simulink model "IEEE14_case"  (R2024b)
settings: Solver=FixedStepAuto  StartTime=0  StopTime=2  FixedStep=1e-7  RelTol=1e-3
values from neighbouring files (symbols this model uses):
  GFL_15_Bva = 0.009    [IEEE14_parameters.m]
  GFL_15_C_bus_pu = 7.179419    [IEEE14_parameters.m]
  GFL_15_f0 = 60    [IEEE14_parameters.m]
  GFL_15_I_id = 691.26967    [IEEE14_parameters.m]
  GFL_15_I_iq = 691.26967    [IEEE14_parameters.m]
  GFL_15_I_od = 45.2207    [IEEE14_parameters.m]
  GFL_15_I_oq = 45.2207    [IEEE14_parameters.m]
  GFL_15_I_pll = 0.78    [IEEE14_parameters.m]
  GFL_15_Kdi = 0.09    [IEEE14_parameters.m]
  GFL_15_Kdo = 0.9    [IEEE14_parameters.m]
  GFL_15_Kqi = 0.09    [IEEE14_parameters.m]
  GFL_15_Kqo = 0.9    [IEEE14_parameters.m]
  GFL_15_Lg_pu = 0.631447    [IEEE14_parameters.m]
  GFL_15_mode = 1    [IEEE14_parameters.m]
  GFL_15_P_id = 3.7166    [IEEE14_parameters.m]
  GFL_15_P_iq = 3.7166    [IEEE14_parameters.m]
  GFL_15_P_od = 0.4798    [IEEE14_parameters.m]
  GFL_15_P_oq = 0.4798    [IEEE14_parameters.m]
  GFL_15_P_pll = 290.42    [IEEE14_parameters.m]
  GFL_15_Qe_ref = 0.2    [IEEE14_parameters.m]
  GFL_15_Rg_pu = 0.024016    [IEEE14_parameters.m]
  GFL_15_Sbase = 1.000000e+4    (= 10000)    [IEEE14_parameters.m]
  GFL_15_Tdi = 0.01    [IEEE14_parameters.m]
  GFL_15_Tdo = 0.2    [IEEE14_parameters.m]
  GFL_15_Tqi = 0.01    [IEEE14_parameters.m]
  GFL_15_Tqo = 0.2    [IEEE14_parameters.m]
  GFL_15_Vbase = 380    [IEEE14_parameters.m]
  GFL_15_Vdc_ref = 1.011475    [IEEE14_parameters.m]
  GFL_15_Vdcbase = 700    [IEEE14_parameters.m]
  GFL_15_vq_ref = 0    [IEEE14_parameters.m]
  GFL_16_Bva = 0.002    [IEEE14_parameters.m]
  GFL_16_C_bus_pu = 7.179419    [IEEE14_parameters.m]
  GFL_16_f0 = 60    [IEEE14_parameters.m]
  GFL_16_I_id = 691.26967    [IEEE14_parameters.m]
  GFL_16_I_iq = 691.26967    [IEEE14_parameters.m]
  GFL_16_I_od = 45.2207    [IEEE14_parameters.m]
  GFL_16_I_oq = 45.2207    [IEEE14_parameters.m]
  GFL_16_I_pll = 0.78    [IEEE14_parameters.m]
  GFL_16_Kdi = 0.05    [IEEE14_parameters.m]
  GFL_16_Kdo = 0.5    [IEEE14_parameters.m]
  GFL_16_Kqi = 0.05    [IEEE14_parameters.m]
  GFL_16_Kqo = 0.5    [IEEE14_parameters.m]
  GFL_16_Lg_pu = 0.631447    [IEEE14_parameters.m]
  GFL_16_mode = 1    [IEEE14_parameters.m]
  GFL_16_P_id = 3.7166    [IEEE14_parameters.m]
  GFL_16_P_iq = 3.7166    [IEEE14_parameters.m]
  GFL_16_P_od = 0.4798    [IEEE14_parameters.m]
  GFL_16_P_oq = 0.4798    [IEEE14_parameters.m]
  GFL_16_P_pll = 290.42    [IEEE14_parameters.m]
  GFL_16_Qe_ref = 0.2    [IEEE14_parameters.m]
  GFL_16_Rg_pu = 0.024016    [IEEE14_parameters.m]
  GFL_16_Sbase = 1.000000e+4    (= 10000)    [IEEE14_parameters.m]
  GFL_16_Tdi = 0.01    [IEEE14_parameters.m]
  GFL_16_Tdo = 0.2    [IEEE14_parameters.m]
  GFL_16_Tqi = 0.01    [IEEE14_parameters.m]
  GFL_16_Tqo = 0.2    [IEEE14_parameters.m]
  GFL_16_Vbase = 380    [IEEE14_parameters.m]
  GFL_16_Vdc_ref = 1.01144    [IEEE14_parameters.m]
  GFL_16_Vdcbase = 700    [IEEE14_parameters.m]
  GFL_16_vq_ref = 0    [IEEE14_parameters.m]
  GFL_17_Bva = 0.002    [IEEE14_parameters.m]
  GFL_17_C_bus_pu = 7.179419    [IEEE14_parameters.m]
  GFL_17_f0 = 60    [IEEE14_parameters.m]
  GFL_17_I_id = 691.26967    [IEEE14_parameters.m]
  GFL_17_I_iq = 691.26967    [IEEE14_parameters.m]
  GFL_17_I_od = 45.2207    [IEEE14_parameters.m]
  GFL_17_I_oq = 45.2207    [IEEE14_parameters.m]
  GFL_17_I_pll = 0.78    [IEEE14_parameters.m]
  GFL_17_Kdi = 0.05    [IEEE14_parameters.m]
  GFL_17_Kdo = 0.5    [IEEE14_parameters.m]
  GFL_17_Kqi = 0.05    [IEEE14_parameters.m]
  GFL_17_Kqo = 0.5    [IEEE14_parameters.m]
  GFL_17_Lg_pu = 0.631447    [IEEE14_parameters.m]
  GFL_17_mode = 1    [IEEE14_parameters.m]
  GFL_17_P_id = 3.7166    [IEEE14_parameters.m]
  GFL_17_P_iq = 3.7166    [IEEE14_parameters.m]
  GFL_17_P_od = 0.4798    [IEEE14_parameters.m]
  GFL_17_P_oq = 0.4798    [IEEE14_parameters.m]
  GFL_17_P_pll = 290.42    [IEEE14_parameters.m]
  GFL_17_Qe_ref = 0.2    [IEEE14_parameters.m]
  GFL_17_Rg_pu = 0.024016    [IEEE14_parameters.m]
  GFL_17_Sbase = 1.000000e+4    (= 10000)    [IEEE14_parameters.m]
  GFL_17_Tdi = 0.01    [IEEE14_parameters.m]
  GFL_17_Tdo = 0.2    [IEEE14_parameters.m]
  GFL_17_Tqi = 0.01    [IEEE14_parameters.m]
  GFL_17_Tqo = 0.2    [IEEE14_parameters.m]
  GFL_17_Vbase = 380    [IEEE14_parameters.m]
  GFL_17_Vdc_ref = 1.011632    [IEEE14_parameters.m]
  GFL_17_Vdcbase = 700    [IEEE14_parameters.m]
  GFL_17_vq_ref = 0    [IEEE14_parameters.m]
  GFL_18_Bva = 0.002    [IEEE14_parameters.m]
  GFL_18_C_bus_pu = 7.179419    [IEEE14_parameters.m]
  GFL_18_f0 = 60    [IEEE14_parameters.m]
  GFL_18_I_id = 691.26967    [IEEE14_parameters.m]
  GFL_18_I_iq = 691.26967    [IEEE14_parameters.m]
  GFL_18_I_od = 45.2207    [IEEE14_parameters.m]
  GFL_18_I_oq = 45.2207    [IEEE14_parameters.m]
  GFL_18_I_pll = 0.78    [IEEE14_parameters.m]
  GFL_18_Kdi = 0.05    [IEEE14_parameters.m]
  GFL_18_Kdo = 0.5    [IEEE14_parameters.m]
  GFL_18_Kqi = 0.05    [IEEE14_parameters.m]
  GFL_18_Kqo = 0.5    [IEEE14_parameters.m]
  GFL_18_Lg_pu = 0.631447    [IEEE14_parameters.m]
  GFL_18_mode = 1    [IEEE14_parameters.m]
  GFL_18_P_id = 3.7166    [IEEE14_parameters.m]
  GFL_18_P_iq = 3.7166    [IEEE14_parameters.m]
  GFL_18_P_od = 0.4798    [IEEE14_parameters.m]
  GFL_18_P_oq = 0.4798    [IEEE14_parameters.m]
  GFL_18_P_pll = 290.42    [IEEE14_parameters.m]
  GFL_18_Qe_ref = 0.2    [IEEE14_parameters.m]
  GFL_18_Rg_pu = 0.024016    [IEEE14_parameters.m]
  GFL_18_Sbase = 1.000000e+4    (= 10000)    [IEEE14_parameters.m]
  GFL_18_Tdi = 0.01    [IEEE14_parameters.m]
  GFL_18_Tdo = 0.2    [IEEE14_parameters.m]
  GFL_18_Tqi = 0.01    [IEEE14_parameters.m]
  GFL_18_Tqo = 0.2    [IEEE14_parameters.m]
  GFL_18_Vbase = 380    [IEEE14_parameters.m]
  GFL_18_Vdc_ref = 1.011572    [IEEE14_parameters.m]
  GFL_18_Vdcbase = 700    [IEEE14_parameters.m]
  GFL_18_vq_ref = 0    [IEEE14_parameters.m]
  ... (+180 more)
(part 18 of 25)

== system IEEE14_case/SG_D_2/d_psi_fd_SG_D_2_block ==
  note: d_psi_fd_SG_D_2 in case14gfl
      | $-\frac{\psi _{\mathrm{fd},\mathrm{SG},D,2}-E_{\mathrm{fd},\mathrm{SG},D,2}+\left(x_{d}-x_{\mathrm{dd}}\right)\,\left(\frac{\frac{\psi _{\mathrm{1d},\mathrm{SG},D,2}\,\left(x_{\mathrm{dd}}-x_{\mathrm{ddd}}\right)}{x_{\mathrm{dd}}-x_{l}}-\psi _{d,\mathrm{SG},D,2}+\frac{\psi _{\mathrm{fd},\mathrm{SG},D,2}\,\left(x_{\mathrm{ddd}}-x_{l}\right)}{x_{\mathrm{dd}}-x_{l}}}{x_{\mathrm{ddd}}}-\frac{\left(x_{\mathrm{dd}}-x_{\mathrm{ddd}}\right)\,\left(\psi _{\mathrm{1d},\mathrm{SG},D,2}-\psi _{\mathrm{fd},\mathrm{SG},D,2}+\frac{\left(x_{\mathrm{dd}}-x_{l}\right)\,\left(\frac{\psi _{\mathrm{1d},\mathrm{SG},D,2}\,\left(x_{\mathrm{dd}}-x_{\mathrm{ddd}}\right)}{x_{\mathrm{dd}}-x_{l}}-\psi _{d,\mathrm{SG},D,2}+\frac{\psi _{\mathrm{fd},\mathrm{SG},D,2}\,\left(x_{\mathrm{ddd}}-x_{l}\right)}{x_{\mathrm{dd}}-x_{l}}\right)}{x_{\mathrm{ddd}}}\right)}{{\left(x_{\mathrm{dd}}-x_{l}\right)}^2}\right)}{T_{\mathrm{dd}}}$
      | Automatically generated on 2025-10-09 21:30:57 .
  State_E_fd_SG_D_2_01a4d : Inport
  State_psi_fd_SG_D_2_2df35 : Inport  Port=2
  State_psi_1d_SG_D_2_84bab : Inport  Port=3
  State_psi_fd_SG_D_2_f521e : Inport  Port=4
  State_psi_1d_SG_D_2_c8d78 : Inport  Port=5
  State_psi_d_SG_D_2_1798b : Inport  Port=6
  State_psi_fd_SG_D_2_82c24 : Inport  Port=7
  State_psi_1d_SG_D_2_e893c : Inport  Port=8
  State_psi_d_SG_D_2_c30ab : Inport  Port=9
  State_psi_fd_SG_D_2_fdcf2 : Inport  Port=10
  Add_3611d : Sum
  Add_4026f : Sum
  Constant_-1_921ca : Constant  Value=-1
  Constant_-1_96da0 : Constant  Value=-1
  Constant_-1_d9610 : Constant  Value=-1
  Constant_2.0_a7520 : Constant  Value=2.0
  Constant_T_dd_003d2 : Constant  Value=T_dd
  Constant_x_d_08df9 : Constant  Value=x_d
  Constant_x_dd_19849 : Constant  Value=x_dd
  Constant_x_dd_47a17 : Constant  Value=x_dd
  Constant_x_dd_565fe : Constant  Value=x_dd
  Constant_x_dd_6360d : Constant  Value=x_dd
  Constant_x_dd_6ee8d : Constant  Value=x_dd
  Constant_x_dd_aa39f : Constant  Value=x_dd
  Constant_x_dd_b6005 : Constant  Value=x_dd
  Constant_x_dd_bbfae : Constant  Value=x_dd
  Constant_x_dd_de48f : Constant  Value=x_dd
  Constant_x_dd_e38b5 : Constant  Value=x_dd
  Constant_x_ddd_0bd47 : Constant  Value=x_ddd
  Constant_x_ddd_846c0 : Constant  Value=x_ddd
  Constant_x_ddd_a248a : Constant  Value=x_ddd
  Constant_x_ddd_a406a : Constant  Value=x_ddd
  Constant_x_ddd_bb480 : Constant  Value=x_ddd
  Constant_x_ddd_ca766 : Constant  Value=x_ddd
  Constant_x_ddd_d5431 : Constant  Value=x_ddd
  Constant_x_l_1bf20 : Constant  Value=x_l
  Constant_x_l_31a91 : Constant  Value=x_l
  Constant_x_l_34653 : Constant  Value=x_l
  Constant_x_l_4eace : Constant  Value=x_l
  Constant_x_l_5aec2 : Constant  Value=x_l
  Constant_x_l_a09cf : Constant  Value=x_l
  Constant_x_l_a2996 : Constant  Value=x_l
  Constant_x_l_ed53a : Constant  Value=x_l
  Divide_1a091 : Product  Inputs=*/
  Divide_320e0 : Product  Inputs=*/
  Divide_4596a : Product  Inputs=*/
  Divide_604a6 : Product  Inputs=*/
  Divide_730ee : Product  Inputs=*/
  Divide_7d69b : Product  Inputs=*/
  Divide_a9374 : Product  Inputs=*/
  Divide_c19ec : Product  Inputs=*/
  Power_098d0 : Math  Operator=pow
  Product_03136 : Product
  Product_07e41 : Product
  Product_25612 : Product
  Product_42463 : Product
  Product_6e0f0 : Product
  Product_8a094 : Product
  Product_90eff : Product
  Product_9aa8a : Product
  Product_a124e : Product
  Product_f461e : Product
  Subtract_04977 : Sum  Inputs=+-
  Subtract_04bd0 : Sum  Inputs=+-
  Subtract_05140 : Sum  Inputs=+-
  Subtract_185b4 : Sum  Inputs=+-
  Subtract_2504d : Sum  Inputs=+-
  Subtract_3f8c2 : Sum  Inputs=+-
  Subtract_446d6 : Sum  Inputs=+-
  Subtract_4df95 : Sum  Inputs=+-
  Subtract_639b5 : Sum  Inputs=+-
  Subtract_64a07 : Sum  Inputs=+-
  Subtract_745c1 : Sum  Inputs=+-
  Subtract_8dab0 : Sum  Inputs=+-
  Subtract_a59fc : Sum  Inputs=+-
  Subtract_ab7fc : Sum  Inputs=+-
  Subtract_cb1a9 : Sum  Inputs=+-
  Subtract_cd5af : Sum  Inputs=+-
  Subtract_cde08 : Sum  Inputs=+-
  Subtract_d078d : Sum  Inputs=+-
  Subtract_ebb1a : Sum  Inputs=+-
  Blockout_d_psi_fd_SG_D_2_ab69d : Outport
  wires:
  Constant_x_dd_bbfae/1 -> Subtract_4df95/1
  Constant_-1_96da0/1 -> Product_42463/1
  Constant_x_l_a09cf/1 -> Subtract_d078d/2
  Divide_1a091/1 -> Add_3611d/1
  Subtract_745c1/1 -> Product_25612/2
  Constant_x_l_1bf20/1 -> Subtract_4df95/2
  Product_25612/1 -> Divide_730ee/1
  State_psi_1d_SG_D_2_c8d78/1 -> Product_42463/2
  Constant_x_dd_b6005/1 -> Subtract_64a07/1
  Product_6e0f0/1 -> Divide_1a091/1
  Constant_x_dd_aa39f/1 -> Subtract_cde08/1
  Constant_x_ddd_d5431/1 -> Subtract_64a07/2
  Constant_x_dd_47a17/1 -> Subtract_8dab0/1
  Product_42463/1 -> Product_f461e/1
  Subtract_64a07/1 -> Product_f461e/2
  State_psi_d_SG_D_2_c30ab/1 -> Add_3611d/2
  Constant_x_ddd_0bd47/1 -> Subtract_745c1/1
  Constant_x_l_31a91/1 -> Subtract_745c1/2
  Product_f461e/1 -> Divide_a9374/1
  Subtract_4df95/1 -> Divide_a9374/2
  State_psi_fd_SG_D_2_82c24/1 -> Product_25612/1
  Subtract_04977/1 -> Product_8a094/2
  Constant_x_dd_565fe/1 -> Subtract_ab7fc/1
  Constant_x_l_34653/1 -> Subtract_ab7fc/2
  Product_07e41/1 -> Product_8a094/1
  Divide_a9374/1 -> Add_4026f/1
  State_psi_d_SG_D_2_1798b/1 -> Add_4026f/2
  Subtract_ab7fc/1 -> Divide_730ee/2
  Constant_x_dd_e38b5/1 -> Subtract_d078d/1
  Constant_x_ddd_a248a/1 -> Subtract_cd5af/1
  Add_4026f/1 -> Subtract_2504d/1
  Divide_730ee/1 -> Subtract_2504d/2
  Constant_-1_d9610/1 -> Product_a124e/1
  Product_9aa8a/1 -> Divide_4596a/1
  State_psi_1d_SG_D_2_e893c/1 -> Product_a124e/2
  Subtract_cde08/1 -> Product_07e41/2
  Constant_x_dd_19849/1 -> Subtract_05140/1
  Divide_4596a/1 -> Subtract_a59fc/2
  Constant_-1_921ca/1 -> Product_07e41/1
  Constant_x_ddd_ca766/1 -> Subtract_05140/2
  Constant_x_ddd_a406a/1 -> Divide_7d69b/2
  Subtract_d078d/1 -> Product_03136/1
  Subtract_2504d/1 -> Product_03136/2
  State_psi_fd_SG_D_2_f521e/1 -> Subtract_ebb1a/2
  Product_a124e/1 -> Product_6e0f0/1
  Subtract_05140/1 -> Product_6e0f0/2
  Constant_2.0_a7520/1 -> Power_098d0/2
  State_psi_1d_SG_D_2_84bab/1 -> Subtract_ebb1a/1
  Constant_x_dd_de48f/1 -> Subtract_639b5/1
  Subtract_cd5af/1 -> Product_9aa8a/2
  Constant_x_l_5aec2/1 -> Subtract_639b5/2
  Constant_x_l_a2996/1 -> Subtract_cd5af/2
  Constant_x_ddd_bb480/1 -> Subtract_cde08/2
  Subtract_8dab0/1 -> Divide_4596a/2
  Product_03136/1 -> Divide_7d69b/1
  Subtract_639b5/1 -> Divide_1a091/2
  State_psi_fd_SG_D_2_fdcf2/1 -> Product_9aa8a/1
  Constant_x_l_4eace/1 -> Subtract_8dab0/2
  Constant_x_dd_6ee8d/1 -> Subtract_185b4/1
  Subtract_ebb1a/1 -> Subtract_04977/1
  Divide_7d69b/1 -> Subtract_04977/2
  Constant_x_l_ed53a/1 -> Subtract_185b4/2
  Subtract_185b4/1 -> Power_098d0/1
  Add_3611d/1 -> Subtract_a59fc/1
  Product_8a094/1 -> Divide_320e0/1
  Power_098d0/1 -> Divide_320e0/2
  Subtract_a59fc/1 -> Divide_c19ec/1
  Constant_x_ddd_846c0/1 -> Divide_c19ec/2
  Constant_x_d_08df9/1 -> Subtract_cb1a9/1
  Constant_x_dd_6360d/1 -> Subtract_cb1a9/2
  Divide_320e0/1 -> Subtract_3f8c2/1
  Divide_c19ec/1 -> Subtract_3f8c2/2
  State_E_fd_SG_D_2_01a4d/1 -> Subtract_446d6/1
  State_psi_fd_SG_D_2_2df35/1 -> Subtract_446d6/2
  Subtract_cb1a9/1 -> Product_90eff/1
  Subtract_3f8c2/1 -> Product_90eff/2
  Subtract_446d6/1 -> Subtract_04bd0/1
  Product_90eff/1 -> Subtract_04bd0/2
  Subtract_04bd0/1 -> Divide_604a6/1
  Constant_T_dd_003d2/1 -> Divide_604a6/2
  Divide_604a6/1 -> Blockout_d_psi_fd_SG_D_2_ab69d/1

== system IEEE14_case/SG_D_2/d_psi_gq_SG_D_2_block ==
  note: d_psi_gq_SG_D_2 in case14gfl
      | $-\frac{\psi _{\mathrm{gq},\mathrm{SG},D,2}+\left(x_{q}-x_{\mathrm{qd}}\right)\,\left(\frac{\psi _{q,\mathrm{SG},D,2}+\frac{\psi _{\mathrm{gq},\mathrm{SG},D,2}\,\left(x_{l}-x_{\mathrm{qdd}}\right)}{x_{l}-x_{\mathrm{qd}}}+\frac{\psi _{\mathrm{kq},\mathrm{SG},D,2}\,\left(x_{\mathrm{qd}}-x_{\mathrm{qdd}}\right)}{x_{l}-x_{\mathrm{qd}}}}{x_{\mathrm{qdd}}}+\frac{\left(x_{\mathrm{qd}}-x_{\mathrm{qdd}}\right)\,\left(\psi _{\mathrm{gq},\mathrm{SG},D,2}+\psi _{\mathrm{kq},\mathrm{SG},D,2}+\frac{\left(x_{l}-x_{\mathrm{qd}}\right)\,\left(\psi _{q,\mathrm{SG},D,2}+\frac{\psi _{\mathrm{gq},\mathrm{SG},D,2}\,\left(x_{l}-x_{\mathrm{qdd}}\right)}{x_{l}-x_{\mathrm{qd}}}+\frac{\psi _{\mathrm{kq},\mathrm{SG},D,2}\,\left(x_{\mathrm{qd}}-x_{\mathrm{qdd}}\right)}{x_{l}-x_{\mathrm{qd}}}\right)}{x_{\mathrm{qdd}}}\right)}{{\left(x_{l}-x_{\mathrm{qd}}\right)}^2}\right)}{T_{\mathrm{qd}}}$
      | Automatically generated on 2025-10-09 21:31:05 .
  State_psi_gq_SG_D_2_f404a : Inport
  State_psi_gq_SG_D_2_79e41 : Inport  Port=2
  State_psi_kq_SG_D_2_229b6 : Inport  Port=3
  State_psi_gq_SG_D_2_41ece : Inport  Port=4
  State_psi_kq_SG_D_2_a4801 : Inport  Port=5
  State_psi_q_SG_D_2_c887c : Inport  Port=6
  State_psi_gq_SG_D_2_c13c7 : Inport  Port=7
  State_psi_kq_SG_D_2_c4824 : Inport  Port=8
  State_psi_q_SG_D_2_400a1 : Inport  Port=9
  Add_2b762 : Sum
  Add_5087b : Sum
  Add_8326a : Sum
  Add_a2ab4 : Sum
  Add_a58ef : Sum
  Add_b9338 : Sum
  Add_bad94 : Sum
  Add_c4542 : Sum
  Add_e5a10 : Sum
  Add_ea486 : Sum
  Add_f567a : Sum
  Add_f8f87 : Sum
  Constant_-1_15cd5 : Constant  Value=-1
  Constant_-1_69318 : Constant  Value=-1
  Constant_-1_75525 : Constant  Value=-1
  Constant_-1_8ad9f : Constant  Value=-1
  Constant_-1_a28c5 : Constant  Value=-1
  Constant_-1_ae299 : Constant  Value=-1
  Constant_-1_b65de : Constant  Value=-1
  Constant_-1_d519c : Constant  Value=-1
  Constant_-1_e17b9 : Constant  Value=-1
  Constant_-1_efabb : Constant  Value=-1
  Constant_2.0_97bc5 : Constant  Value=2.0
  Constant_T_qd_686ff : Constant  Value=T_qd
  Constant_x_l_09c66 : Constant  Value=x_l
  Constant_x_l_1d2f7 : Constant  Value=x_l
  Constant_x_l_4d818 : Constant  Value=x_l
  Constant_x_l_57d53 : Constant  Value=x_l
  Constant_x_l_74c75 : Constant  Value=x_l
  Constant_x_l_b1845 : Constant  Value=x_l
  Constant_x_l_ba1dd : Constant  Value=x_l
  Constant_x_l_bbcc9 : Constant  Value=x_l
  Constant_x_q_f52e3 : Constant  Value=x_q
  Constant_x_qd_2dcf1 : Constant  Value=x_qd
  Constant_x_qd_3806a : Constant  Value=x_qd
  Constant_x_qd_3a214 : Constant  Value=x_qd
  Constant_x_qd_46c49 : Constant  Value=x_qd
  Constant_x_qd_478ae : Constant  Value=x_qd
  Constant_x_qd_63b72 : Constant  Value=x_qd
  Constant_x_qd_820ca : Constant  Value=x_qd
  Constant_x_qd_9db90 : Constant  Value=x_qd
  Constant_x_qd_b7357 : Constant  Value=x_qd
  Constant_x_qd_e39da : Constant  Value=x_qd
  Constant_x_qdd_17fcd : Constant  Value=x_qdd
  Constant_x_qdd_4d231 : Constant  Value=x_qdd
  Constant_x_qdd_b2109 : Constant  Value=x_qdd
  Constant_x_qdd_b62fd : Constant  Value=x_qdd
  Constant_x_qdd_bd892 : Constant  Value=x_qdd
  Constant_x_qdd_c0bf7 : Constant  Value=x_qdd
  Constant_x_qdd_c1908 : Constant  Value=x_qdd
  Divide_500ab : Product  Inputs=*/
  Divide_5990b : Product  Inputs=*/
  Divide_60d9c : Product  Inputs=*/
  Divide_8a86b : Product  Inputs=*/
  Divide_97166 : Product  Inputs=*/
  Divide_a2283 : Product  Inputs=*/
  Divide_d0dda : Product  Inputs=*/
  Divide_f3509 : Product  Inputs=*/
  Power_100eb : Math  Operator=pow
  Product_2ab9d : Product
  Product_2ef50 : Product
  Product_52ea3 : Product
  Product_6e281 : Product
  Product_94fc7 : Product
  Product_9831b : Product
  Product_9d28f : Product
  Product_a2030 : Product
  Product_aac4e : Product
  Product_ac00d : Product
  Product_acce0 : Product
  Product_b35c4 : Product
  Product_b7c07 : Product
  Product_c4254 : Product
  Product_e9acb : Product
  Product_ef741 : Product
  Product_f98fe : Product
  Subtract_18ab3 : Sum  Inputs=+-
  Subtract_23d70 : Sum  Inputs=+-
  Subtract_3e5e5 : Sum  Inputs=+-
  Subtract_52e88 : Sum  Inputs=+-
  Subtract_71078 : Sum  Inputs=+-
  Subtract_881b9 : Sum  Inputs=+-
  Subtract_c6265 : Sum  Inputs=+-
  Subtract_cf1d4 : Sum  Inputs=+-
  Blockout_d_psi_gq_SG_D_2_f3eae : Outport
  wires:
  Constant_x_l_b1845/1 -> Product_52ea3/2
  Constant_x_l_57d53/1 -> Product_acce0/2
  Constant_x_qd_2dcf1/1 -> Subtract_881b9/1
  Constant_x_l_ba1dd/1 -> Product_a2030/2
  Constant_x_qdd_17fcd/1 -> Subtract_71078/2
  Constant_-1_ae299/1 -> Product_b35c4/1
  Constant_-1_e17b9/1 -> Product_aac4e/1
  State_psi_gq_SG_D_2_79e41/1 -> Add_8326a/1
  Constant_x_qdd_c0bf7/1 -> Subtract_881b9/2
  Constant_x_qd_b7357/1 -> Subtract_71078/1
  Constant_x_l_bbcc9/1 -> Product_b35c4/2
  Constant_x_l_09c66/1 -> Product_aac4e/2
  Product_b35c4/1 -> Add_c4542/1
  Product_aac4e/1 -> Add_2b762/1
  Constant_x_l_74c75/1 -> Product_94fc7/2
  Constant_x_l_1d2f7/1 -> Product_ac00d/2
  Constant_x_qd_3806a/1 -> Add_c4542/2
  Constant_x_qdd_bd892/1 -> Add_2b762/2
  Constant_-1_15cd5/1 -> Product_94fc7/1
  Constant_x_qd_820ca/1 -> Add_ea486/2
  Constant_x_qdd_b62fd/1 -> Add_a58ef/2
  State_psi_gq_SG_D_2_41ece/1 -> Product_2ef50/1
  Add_c4542/1 -> Divide_500ab/2
  Add_2b762/1 -> Product_2ef50/2
  Constant_x_qd_46c49/1 -> Subtract_23d70/2
  Product_94fc7/1 -> Add_5087b/1
  Constant_x_qd_3a214/1 -> Add_5087b/2
  State_psi_kq_SG_D_2_a4801/1 -> Product_ef741/1
  Divide_97166/1 -> Subtract_cf1d4/1
  Subtract_881b9/1 -> Product_ef741/2
  Product_2ef50/1 -> Divide_97166/1
  Add_5087b/1 -> Divide_97166/2
  Add_e5a10/1 -> Product_9d28f/2
  Product_ef741/1 -> Divide_500ab/1
  Constant_-1_8ad9f/1 -> Product_ac00d/1
  Divide_500ab/1 -> Subtract_cf1d4/2
  Constant_-1_69318/1 -> Product_52ea3/1
  Constant_-1_a28c5/1 -> Product_acce0/1
  Product_ac00d/1 -> Add_bad94/1
  Constant_x_qdd_4d231/1 -> Subtract_52e88/2
  Constant_x_qd_63b72/1 -> Add_bad94/2
  Subtract_cf1d4/1 -> Add_e5a10/1
  Constant_-1_b65de/1 -> Product_a2030/1
  State_psi_q_SG_D_2_c887c/1 -> Add_e5a10/2
  Product_52ea3/1 -> Add_ea486/1
  Product_acce0/1 -> Add_a58ef/1
  Constant_-1_75525/1 -> Product_9831b/1
  Product_9d28f/1 -> Divide_d0dda/1
  Constant_x_l_4d818/1 -> Product_9831b/2
  Product_2ab9d/1 -> Add_f567a/2
  Constant_x_qd_e39da/1 -> Subtract_52e88/1
  Add_bad94/1 -> Product_9d28f/1
  State_psi_gq_SG_D_2_c13c7/1 -> Product_e9acb/1
  Add_ea486/1 -> Divide_f3509/2
  Add_a58ef/1 -> Product_e9acb/2
  Product_9831b/1 -> Add_b9338/1
  Constant_x_qd_478ae/1 -> Add_b9338/2
  State_psi_kq_SG_D_2_c4824/1 -> Product_f98fe/1
  Subtract_52e88/1 -> Product_f98fe/2
  Divide_f3509/1 -> Subtract_18ab3/2
  State_psi_kq_SG_D_2_229b6/1 -> Add_8326a/2
  Product_f98fe/1 -> Divide_f3509/1
  Constant_x_qdd_c1908/1 -> Divide_d0dda/2
  Product_e9acb/1 -> Divide_8a86b/1
  Add_b9338/1 -> Divide_8a86b/2
  Constant_-1_d519c/1 -> Product_6e281/1
  Subtract_71078/1 -> Product_6e281/2
  Add_8326a/1 -> Subtract_3e5e5/1
  Divide_d0dda/1 -> Subtract_3e5e5/2
  Product_a2030/1 -> Add_a2ab4/1
  Constant_x_qd_9db90/1 -> Add_a2ab4/2
  Divide_8a86b/1 -> Subtract_18ab3/1
  Product_6e281/1 -> Product_b7c07/1
  Subtract_3e5e5/1 -> Product_b7c07/2
  Add_a2ab4/1 -> Power_100eb/1
  Constant_2.0_97bc5/1 -> Power_100eb/2
  Subtract_18ab3/1 -> Add_f8f87/1
  State_psi_q_SG_D_2_400a1/1 -> Add_f8f87/2
  Product_b7c07/1 -> Divide_a2283/1
  Power_100eb/1 -> Divide_a2283/2
  Add_f8f87/1 -> Divide_60d9c/1
  Constant_x_qdd_b2109/1 -> Divide_60d9c/2
  Constant_x_q_f52e3/1 -> Subtract_23d70/1
  Divide_a2283/1 -> Subtract_c6265/1
  Divide_60d9c/1 -> Subtract_c6265/2
  Divide_5990b/1 -> Blockout_d_psi_gq_SG_D_2_f3eae/1
  Constant_-1_efabb/1 -> Product_c4254/1
  State_psi_gq_SG_D_2_f404a/1 -> Product_c4254/2
  Subtract_23d70/1 -> Product_2ab9d/1
  Subtract_c6265/1 -> Product_2ab9d/2
  Product_c4254/1 -> Add_f567a/1
  Add_f567a/1 -> Divide_5990b/1
  Constant_T_qd_686ff/1 -> Divide_5990b/2

== system IEEE14_case/SG_D_2/d_psi_kq_SG_D_2_block ==
  note: d_psi_kq_SG_D_2 in case14gfl
      | $-\frac{\psi _{\mathrm{gq},\mathrm{SG},D,2}+\psi _{\mathrm{kq},\mathrm{SG},D,2}+\frac{\left(x_{l}-x_{\mathrm{qd}}\right)\,\left(\psi _{q,\mathrm{SG},D,2}+\frac{\psi _{\mathrm{gq},\mathrm{SG},D,2}\,\left(x_{l}-x_{\mathrm{qdd}}\right)}{x_{l}-x_{\mathrm{qd}}}+\frac{\psi _{\mathrm{kq},\mathrm{SG},D,2}\,\left(x_{\mathrm{qd}}-x_{\mathrm{qdd}}\right)}{x_{l}-x_{\mathrm{qd}}}\right)}{x_{\mathrm{qdd}}}}{T_{\mathrm{qdd}}}$
      | Automatically generated on 2025-10-09 21:31:07 .
  State_psi_gq_SG_D_2_f92a1 : Inport
  State_psi_kq_SG_D_2_f7bb1 : Inport  Port=2
  State_psi_gq_SG_D_2_cbe5c : Inport  Port=3
  State_psi_kq_SG_D_2_18fe7 : Inport  Port=4
  State_psi_q_SG_D_2_cfb7c : Inport  Port=5
  Add_2481c : Sum
  Add_2fdb3 : Sum
  Add_3b297 : Sum
  Add_3ce2d : Sum
  Add_7fdac : Sum
  Add_eb29d : Sum
  Constant_-1_13a81 : Constant  Value=-1
  Constant_-1_44d95 : Constant  Value=-1
  Constant_-1_6f5fa : Constant  Value=-1
  Constant_-1_e2c15 : Constant  Value=-1
  Constant_-1_e723b : Constant  Value=-1
  Constant_T_qdd_cc972 : Constant  Value=T_qdd
  Constant_x_l_9fa0f : Constant  Value=x_l
  Constant_x_l_c253f : Constant  Value=x_l
  Constant_x_l_dc0da : Constant  Value=x_l
  Constant_x_l_e4987 : Constant  Value=x_l
  Constant_x_qd_849ec : Constant  Value=x_qd
  Constant_x_qd_9b99b : Constant  Value=x_qd
  Constant_x_qd_a0e14 : Constant  Value=x_qd
  Constant_x_qd_a3048 : Constant  Value=x_qd
  Constant_x_qdd_317d9 : Constant  Value=x_qdd
  Constant_x_qdd_60f94 : Constant  Value=x_qdd
  Constant_x_qdd_dadcf : Constant  Value=x_qdd
  Divide_2b384 : Product  Inputs=*/
  Divide_80f05 : Product  Inputs=*/
  Divide_847ec : Product  Inputs=*/
  Divide_c48ac : Product  Inputs=*/
  Product_39d4f : Product
  Product_45e1e : Product
  Product_6192a : Product
  Product_87c85 : Product
  Product_998de : Product
  Product_a46e6 : Product
  Product_adb8e : Product
  Product_e290e : Product
  Subtract_b28c8 : Sum  Inputs=+-
  Subtract_b9688 : Sum  Inputs=+-
  Subtract_d8af5 : Sum  Inputs=+-
  Blockout_d_psi_kq_SG_D_2_03e6e : Outport
  wires:
  State_psi_kq_SG_D_2_f7bb1/1 -> Subtract_b9688/2
  Constant_-1_44d95/1 -> Product_6192a/1
  Constant_-1_e2c15/1 -> Product_e290e/1
  Constant_x_l_e4987/1 -> Product_e290e/2
  Constant_x_qdd_317d9/1 -> Add_2fdb3/2
  Constant_x_l_c253f/1 -> Product_6192a/2
  Constant_x_qd_a3048/1 -> Subtract_b28c8/1
  Constant_T_qdd_cc972/1 -> Divide_c48ac/2
  Constant_-1_13a81/1 -> Product_45e1e/1
  Product_e290e/1 -> Add_2fdb3/1
  Constant_x_qdd_dadcf/1 -> Subtract_b28c8/2
  Constant_x_l_9fa0f/1 -> Product_45e1e/2
  Divide_c48ac/1 -> Blockout_d_psi_kq_SG_D_2_03e6e/1
  State_psi_gq_SG_D_2_cbe5c/1 -> Product_39d4f/1
  Add_2fdb3/1 -> Product_39d4f/2
  Product_6192a/1 -> Add_2481c/1
  Constant_x_qd_849ec/1 -> Add_2481c/2
  Product_a46e6/1 -> Divide_2b384/1
  State_psi_kq_SG_D_2_18fe7/1 -> Product_998de/1
  Subtract_b28c8/1 -> Product_998de/2
  Product_45e1e/1 -> Add_3ce2d/1
  Constant_x_qd_9b99b/1 -> Add_3ce2d/2
  Product_998de/1 -> Divide_80f05/1
  Product_39d4f/1 -> Divide_847ec/1
  Add_2481c/1 -> Divide_847ec/2
  Add_3ce2d/1 -> Divide_80f05/2
  State_psi_q_SG_D_2_cfb7c/1 -> Add_7fdac/2
  Constant_-1_e723b/1 -> Product_87c85/1
  Constant_x_l_dc0da/1 -> Product_87c85/2
  Divide_847ec/1 -> Subtract_d8af5/1
  Divide_80f05/1 -> Subtract_d8af5/2
  Product_87c85/1 -> Add_3b297/1
  Constant_x_qd_a0e14/1 -> Add_3b297/2
  Subtract_d8af5/1 -> Add_7fdac/1
  Constant_x_qdd_60f94/1 -> Divide_2b384/2
  Constant_-1_6f5fa/1 -> Product_adb8e/1
  State_psi_gq_SG_D_2_f92a1/1 -> Product_adb8e/2
  Add_3b297/1 -> Product_a46e6/1
  Add_7fdac/1 -> Product_a46e6/2
  Product_adb8e/1 -> Subtract_b9688/1
  Subtract_b9688/1 -> Add_eb29d/1
  Divide_2b384/1 -> Add_eb29d/2
  Add_eb29d/1 -> Divide_c48ac/1

== system IEEE14_case/SG_D_2/d_psi_q_SG_D_2_block ==
  note: d_psi_q_SG_D_2 in case14gfl
      | $2\,\pi \,f_{0}\,\left(v_{d,\mathrm{SG},D,2}\,\cos\left(\theta _{\mathrm{SG},D,2}\right)+v_{q,\mathrm{SG},D,2}\,\sin\left(\theta _{\mathrm{SG},D,2}\right)-\frac{R_{a}\,\left(\psi _{q,\mathrm{SG},D,2}+\frac{\psi _{\mathrm{gq},\mathrm{SG},D,2}\,\left(x_{l}-x_{\mathrm{qdd}}\right)}{x_{l}-x_{\mathrm{qd}}}+\frac{\psi _{\mathrm{kq},\mathrm{SG},D,2}\,\left(x_{\mathrm{qd}}-x_{\mathrm{qdd}}\right)}{x_{l}-x_{\mathrm{qd}}}\right)}{x_{\mathrm{qdd}}}-\frac{\psi _{d,\mathrm{SG},D,2}\,w_{\mathrm{SG},D,2}}{2\,f_{0}\,\pi }\right)$
      | Automatically generated on 2025-10-09 21:30:53 .
  State_psi_gq_SG_D_2_7a17f : Inport
  State_psi_kq_SG_D_2_3a32d : Inport  Port=2
  State_psi_q_SG_D_2_b05c7 : Inport  Port=3
  Input_v_d_SG_D_2_1b10e : Inport  Port=4
  State_theta_SG_D_2_ba654 : Inport  Port=5
  Input_v_q_SG_D_2_876cf : Inport  Port=6
  State_theta_SG_D_2_5db71 : Inport  Port=7
  State_psi_d_SG_D_2_4f2c3 : Inport  Port=8
  State_w_SG_D_2_ecb88 : Inport  Port=9
  Add_04e7d : Sum
  Add_1a74e : Sum
  Add_788e4 : Sum
  Add_bf7d8 : Sum
  Add_e6fa3 : Sum
  Constant_-1_35839 : Constant  Value=-1
  Constant_-1_49f51 : Constant  Value=-1
  Constant_-1_facd6 : Constant  Value=-1
  Constant_-2.0_3d548 : Constant  Value=-2.0
  Constant_2.0_6b09a : Constant  Value=2.0
  Constant_R_a_9db04 : Constant  Value=R_a
  Constant_f0_153f0 : Constant  Value=f0
  Constant_f0_f7162 : Constant  Value=f0
  Constant_pi_a6f6d : Constant  Value=pi
  Constant_pi_c7144 : Constant  Value=pi
  Constant_x_l_0338e : Constant  Value=x_l
  Constant_x_l_9d415 : Constant  Value=x_l
  Constant_x_l_d5d7c : Constant  Value=x_l
  Constant_x_qd_1b162 : Constant  Value=x_qd
  Constant_x_qd_c48bf : Constant  Value=x_qd
  Constant_x_qd_c7134 : Constant  Value=x_qd
  Constant_x_qdd_09f60 : Constant  Value=x_qdd
  Constant_x_qdd_296de : Constant  Value=x_qdd
  Constant_x_qdd_5a348 : Constant  Value=x_qdd
  Divide_118c2 : Product  Inputs=*/
  Divide_c202d : Product  Inputs=*/
  Divide_d2c50 : Product  Inputs=*/
  Divide_e1b55 : Product  Inputs=*/
  MathFunc_cos_359bc : Trigonometry  Operator=cos
  MathFunc_sin_6875e : Trigonometry
  Product_097c8 : Product
  Product_2c956 : Product
  Product_55d7c : Product
  Product_5a829 : Product
  Product_5cc17 : Product
  Product_7fbb7 : Product
  Product_86d9b : Product
  Product_9233d : Product
  Product_9e59a : Product
  Product_a2ff4 : Product
  Product_a7b7f : Product
  Product_b027a : Product
  Product_e8368 : Product
  Product_efeb8 : Product
  Subtract_30749 : Sum  Inputs=+-
  Subtract_4455b : Sum  Inputs=+-
  Subtract_4bbc0 : Sum  Inputs=+-
  Subtract_d97d7 : Sum  Inputs=+-
  Blockout_d_psi_q_SG_D_2_a5b60 : Outport
  wires:
  Constant_x_qdd_09f60/1 -> Subtract_4bbc0/2
  Constant_x_l_0338e/1 -> Product_e8368/2
  Constant_-1_35839/1 -> Product_a7b7f/1
  Constant_x_l_9d415/1 -> Product_a7b7f/2
  Product_a7b7f/1 -> Add_04e7d/1
  Constant_pi_c7144/1 -> Product_9e59a/2
  State_psi_gq_SG_D_2_7a17f/1 -> Product_5cc17/1
  Constant_x_l_d5d7c/1 -> Product_5a829/2
  State_w_SG_D_2_ecb88/1 -> Product_a2ff4/2
  Constant_x_qd_1b162/1 -> Add_1a74e/2
  Constant_x_qdd_296de/1 -> Add_04e7d/2
  Constant_2.0_6b09a/1 -> Product_9e59a/1
  Constant_-1_facd6/1 -> Product_5a829/1
  Constant_x_qd_c7134/1 -> Subtract_4bbc0/1
  Constant_-1_49f51/1 -> Product_e8368/1
  State_psi_q_SG_D_2_b05c7/1 -> Add_bf7d8/2
  Add_04e7d/1 -> Product_5cc17/2
  Product_9e59a/1 -> Product_9233d/1
  Product_5a829/1 -> Add_788e4/1
  Constant_pi_a6f6d/1 -> Product_2c956/2
  Constant_f0_f7162/1 -> Product_9233d/2
  Constant_x_qd_c48bf/1 -> Add_788e4/2
  State_psi_kq_SG_D_2_3a32d/1 -> Product_097c8/1
  Subtract_4bbc0/1 -> Product_097c8/2
  Product_e8368/1 -> Add_1a74e/1
  Input_v_q_SG_D_2_876cf/1 -> Product_86d9b/1
  Product_5cc17/1 -> Divide_c202d/1
  Product_9233d/1 -> Divide_e1b55/2
  Add_788e4/1 -> Divide_c202d/2
  Product_097c8/1 -> Divide_118c2/1
  Add_1a74e/1 -> Divide_118c2/2
  Divide_c202d/1 -> Subtract_4455b/1
  State_theta_SG_D_2_ba654/1 -> MathFunc_cos_359bc/1
  Divide_118c2/1 -> Subtract_4455b/2
  Subtract_4455b/1 -> Add_bf7d8/1
  MathFunc_cos_359bc/1 -> Product_efeb8/2
  Constant_R_a_9db04/1 -> Product_55d7c/1
  Add_bf7d8/1 -> Product_55d7c/2
  State_theta_SG_D_2_5db71/1 -> MathFunc_sin_6875e/1
  Product_55d7c/1 -> Divide_d2c50/1
  Product_2c956/1 -> Product_7fbb7/1
  Product_86d9b/1 -> Subtract_d97d7/2
  Constant_x_qdd_5a348/1 -> Divide_d2c50/2
  Input_v_d_SG_D_2_1b10e/1 -> Product_efeb8/1
  Add_e6fa3/1 -> Product_b027a/2
  Divide_d2c50/1 -> Subtract_30749/1
  Product_efeb8/1 -> Subtract_30749/2
  MathFunc_sin_6875e/1 -> Product_86d9b/2
  Product_b027a/1 -> Blockout_d_psi_q_SG_D_2_a5b60/1
  State_psi_d_SG_D_2_4f2c3/1 -> Product_a2ff4/1
  Constant_-2.0_3d548/1 -> Product_2c956/1
  Product_7fbb7/1 -> Product_b027a/1
  Subtract_30749/1 -> Subtract_d97d7/1
  Product_a2ff4/1 -> Divide_e1b55/1
  Constant_f0_153f0/1 -> Product_7fbb7/2
  Subtract_d97d7/1 -> Add_e6fa3/1
  Divide_e1b55/1 -> Add_e6fa3/2

== system IEEE14_case/SG_D_2/d_theta_SG_D_2_block ==
  note: d_theta_SG_D_2 in case14gfl
      | $w_{\mathrm{SG},D,2}-2\,\pi \,f_{0}$
      | Automatically generated on 2025-10-09 21:31:14 .
  State_w_SG_D_2_44e1a : Inport
  Add_5fae3 : Sum
  Constant_-2.0_72754 : Constant  Value=-2.0
  Constant_f0_c2c99 : Constant  Value=f0
  Constant_pi_62341 : Constant  Value=pi
  Product_000eb : Product
  Product_08167 : Product
  Blockout_d_theta_SG_D_2_e87fa : Outport
  wires:
  Constant_-2.0_72754/1 -> Product_08167/1
  Constant_pi_62341/1 -> Product_08167/2
  Add_5fae3/1 -> Blockout_d_theta_SG_D_2_e87fa/1
  Product_08167/1 -> Product_000eb/1
  Constant_f0_c2c99/1 -> Product_000eb/2
  Product_000eb/1 -> Add_5fae3/1
  State_w_SG_D_2_44e1a/1 -> Add_5fae3/2

== system IEEE14_case/SG_D_2/d_w_SG_D_2_block ==
  note: d_w_SG_D_2 in case14gfl
      | $\frac{2\,\pi \,T_{m,\mathrm{SG},D,2}\,f_{0}-D\,\left(w_{\mathrm{SG},D,2}-2\,\pi \,f_{0}\right)+2\,\pi \,f_{0}\,\left(\frac{\psi _{d,\mathrm{SG},D,2}\,\left(\psi _{q,\mathrm{SG},D,2}+\frac{\psi _{\mathrm{gq},\mathrm{SG},D,2}\,\left(x_{l}-x_{\mathrm{qdd}}\right)}{x_{l}-x_{\mathrm{qd}}}+\frac{\psi _{\mathrm{kq},\mathrm{SG},D,2}\,\left(x_{\mathrm{qd}}-x_{\mathrm{qdd}}\right)}{x_{l}-x_{\mathrm{qd}}}\right)}{x_{\mathrm{qdd}}}+\frac{\psi _{q,\mathrm{SG},D,2}\,\left(\frac{\psi _{\mathrm{1d},\mathrm{SG},D,2}\,\left(x_{\mathrm{dd}}-x_{\mathrm{ddd}}\right)}{x_{\mathrm{dd}}-x_{l}}-\psi _{d,\mathrm{SG},D,2}+\frac{\psi _{\mathrm{fd},\mathrm{SG},D,2}\,\left(x_{\mathrm{ddd}}-x_{l}\right)}{x_{\mathrm{dd}}-x_{l}}\right)}{x_{\mathrm{ddd}}}\right)}{2\,H}$
      | Automatically generated on 2025-10-09 21:31:12 .
  State_w_SG_D_2_04eee : Inport
  State_T_m_SG_D_2_0748f : Inport  Port=2
  State_psi_d_SG_D_2_6ae82 : Inport  Port=3
  State_psi_gq_SG_D_2_fb75f : Inport  Port=4
  State_psi_kq_SG_D_2_19d78 : Inport  Port=5
  State_psi_q_SG_D_2_03373 : Inport  Port=6
  State_psi_q_SG_D_2_8635e : Inport  Port=7
  State_psi_1d_SG_D_2_3458c : Inport  Port=8
  State_psi_d_SG_D_2_d3800 : Inport  Port=9
  State_psi_fd_SG_D_2_b728a : Inport  Port=10
  Add_273e9 : Sum
  Add_5171a : Sum
  Add_715a6 : Sum
  Add_ab984 : Sum
  Add_c2013 : Sum
  Add_daafc : Sum
  Add_f75dd : Sum
  Add_fcdb9 : Sum
  Constant_-1_09c0e : Constant  Value=-1
  Constant_-1_28d1d : Constant  Value=-1
  Constant_-1_3b28a : Constant  Value=-1
  Constant_-1_5afab : Constant  Value=-1
  Constant_-1_b9d9f : Constant  Value=-1
  Constant_-1_ef6a3 : Constant  Value=-1
  Constant_-2.0_f88f3 : Constant  Value=-2.0
  Constant_2.0_379f0 : Constant  Value=2.0
  Constant_2.0_47047 : Constant  Value=2.0
  Constant_2.0_c1cc6 : Constant  Value=2.0
  Constant_D_8112f : Constant  Value=D
  Constant_H_bef7b : Constant  Value=H
  Constant_f0_2127e : Constant  Value=f0
  Constant_f0_c9729 : Constant  Value=f0
  Constant_f0_f003f : Constant  Value=f0
  Constant_pi_73b2a : Constant  Value=pi
  Constant_pi_84408 : Constant  Value=pi
  Constant_pi_eaa3b : Constant  Value=pi
  Constant_x_dd_05788 : Constant  Value=x_dd
  Constant_x_dd_171a6 : Constant  Value=x_dd
  Constant_x_dd_eae0d : Constant  Value=x_dd
  Constant_x_ddd_33146 : Constant  Value=x_ddd
  Constant_x_ddd_78f1e : Constant  Value=x_ddd
  Constant_x_ddd_c2439 : Constant  Value=x_ddd
  Constant_x_l_425c2 : Constant  Value=x_l
  Constant_x_l_788cd : Constant  Value=x_l
  Constant_x_l_7d8cc : Constant  Value=x_l
  Constant_x_l_938e0 : Constant  Value=x_l
  Constant_x_l_a4da0 : Constant  Value=x_l
  Constant_x_l_b46fa : Constant  Value=x_l
  Constant_x_qd_379d5 : Constant  Value=x_qd
  Constant_x_qd_4b3de : Constant  Value=x_qd
  Constant_x_qd_f22c5 : Constant  Value=x_qd
  Constant_x_qdd_0c78e : Constant  Value=x_qdd
  Constant_x_qdd_45266 : Constant  Value=x_qdd
  Constant_x_qdd_63602 : Constant  Value=x_qdd
  Divide_0cd8d : Product  Inputs=*/
  Divide_2b866 : Product  Inputs=*/
  Divide_3bd14 : Product  Inputs=*/
  Divide_5f5cf : Product  Inputs=*/
  Divide_67709 : Product  Inputs=*/
  Divide_714fc : Product  Inputs=*/
  Divide_c5a16 : Product  Inputs=*/
  Product_0b5d5 : Product
  Product_1e49f : Product
  Product_30f4f : Product
  Product_342b7 : Product
  Product_3ef8a : Product
  Product_4a403 : Product
  Product_5a295 : Product
  Product_5a5f0 : Product
  Product_814fc : Product
  Product_8423e : Product
  Product_8afa9 : Product
  Product_b7481 : Product
  Product_baf2a : Product
  Product_bc693 : Product
  Product_d0595 : Product
  Product_d448e : Product
  Product_dec45 : Product
  Product_e288b : Product
  Product_e5e84 : Product
  Product_eccf3 : Product
  Product_f3747 : Product
  Product_fe42d : Product
  Subtract_1b812 : Sum  Inputs=+-
  Subtract_200d5 : Sum  Inputs=+-
  Subtract_4fc82 : Sum  Inputs=+-
  Subtract_525a6 : Sum  Inputs=+-
  Subtract_8fa5a : Sum  Inputs=+-
  Subtract_a3e8f : Sum  Inputs=+-
  Subtract_bff4c : Sum  Inputs=+-
  Subtract_f038b : Sum  Inputs=+-
  Blockout_d_w_SG_D_2_78b05 : Outport
  wires:
  Constant_x_qd_4b3de/1 -> Subtract_bff4c/1
  Constant_-1_09c0e/1 -> Product_342b7/1
  Constant_-1_ef6a3/1 -> Product_8423e/1
  Constant_x_qdd_45266/1 -> Subtract_bff4c/2
  Subtract_8fa5a/1 -> Divide_3bd14/2
  Constant_x_l_a4da0/1 -> Product_342b7/2
  Constant_x_l_788cd/1 -> Product_8423e/2
  Product_342b7/1 -> Add_ab984/1
  Product_8423e/1 -> Add_c2013/1
  Constant_x_l_b46fa/1 -> Subtract_525a6/2
  Constant_x_l_425c2/1 -> Product_f3747/2
  Constant_x_ddd_c2439/1 -> Divide_0cd8d/2
  Subtract_200d5/1 -> Product_fe42d/2
  Constant_x_qd_f22c5/1 -> Add_ab984/2
  Constant_x_qdd_63602/1 -> Add_c2013/2
  Constant_-1_b9d9f/1 -> Product_f3747/1
  State_psi_d_SG_D_2_6ae82/1 -> Product_1e49f/2
  Constant_-1_28d1d/1 -> Product_b7481/1
  State_w_SG_D_2_04eee/1 -> Add_715a6/2
  Product_f3747/1 -> Add_273e9/1
  State_psi_1d_SG_D_2_3458c/1 -> Product_b7481/2
  Constant_x_dd_05788/1 -> Subtract_1b812/1
  Divide_c5a16/1 -> Subtract_f038b/1
  Subtract_bff4c/1 -> Product_e288b/2
  Constant_x_ddd_78f1e/1 -> Subtract_1b812/2
  State_psi_gq_SG_D_2_fb75f/1 -> Product_bc693/1
  Add_ab984/1 -> Divide_5f5cf/2
  State_psi_d_SG_D_2_d3800/1 -> Add_5171a/2
  Add_c2013/1 -> Product_bc693/2
  Constant_x_qd_379d5/1 -> Add_273e9/2
  State_psi_kq_SG_D_2_19d78/1 -> Product_e288b/1
  Product_b7481/1 -> Product_baf2a/1
  Subtract_1b812/1 -> Product_baf2a/2
  Constant_pi_84408/1 -> Product_814fc/2
  Constant_x_dd_eae0d/1 -> Subtract_525a6/1
  Constant_x_ddd_33146/1 -> Subtract_200d5/1
  Constant_x_l_7d8cc/1 -> Subtract_200d5/2
  Product_bc693/1 -> Divide_c5a16/1
  Add_273e9/1 -> Divide_c5a16/2
  Add_daafc/1 -> Product_5a5f0/2
  Product_e288b/1 -> Divide_5f5cf/1
  Constant_pi_73b2a/1 -> Product_0b5d5/2
  Product_baf2a/1 -> Divide_714fc/1
  Subtract_525a6/1 -> Divide_714fc/2
  State_psi_fd_SG_D_2_b728a/1 -> Product_fe42d/1
  Divide_714fc/1 -> Add_5171a/1
  Constant_x_dd_171a6/1 -> Subtract_8fa5a/1
  Constant_x_l_938e0/1 -> Subtract_8fa5a/2
  Divide_5f5cf/1 -> Subtract_f038b/2
  Product_fe42d/1 -> Divide_3bd14/1
  Constant_-1_3b28a/1 -> Product_1e49f/1
  Constant_-2.0_f88f3/1 -> Product_0b5d5/1
  Subtract_f038b/1 -> Add_daafc/1
  Subtract_a3e8f/1 -> Product_dec45/2
  State_psi_q_SG_D_2_03373/1 -> Add_daafc/2
  Constant_D_8112f/1 -> Product_d448e/2
  Add_5171a/1 -> Subtract_a3e8f/1
  Divide_3bd14/1 -> Subtract_a3e8f/2
  Product_0b5d5/1 -> Product_d0595/1
  Constant_f0_f003f/1 -> Product_d0595/2
  Constant_2.0_379f0/1 -> Product_814fc/1
  Product_1e49f/1 -> Product_5a5f0/1
  State_psi_q_SG_D_2_8635e/1 -> Product_dec45/1
  Constant_-1_5afab/1 -> Product_d448e/1
  Product_d0595/1 -> Add_715a6/1
  Product_814fc/1 -> Product_4a403/1
  State_T_m_SG_D_2_0748f/1 -> Product_4a403/2
  Constant_2.0_c1cc6/1 -> Product_e5e84/1
  Constant_pi_eaa3b/1 -> Product_e5e84/2
  Product_5a5f0/1 -> Divide_67709/1
  Constant_x_qdd_0c78e/1 -> Divide_67709/2
  Product_dec45/1 -> Divide_0cd8d/1
  Product_d448e/1 -> Product_eccf3/1
  Add_715a6/1 -> Product_eccf3/2
  Product_4a403/1 -> Product_30f4f/1
  Constant_f0_c9729/1 -> Product_30f4f/2
  Product_e5e84/1 -> Product_3ef8a/1
  Constant_f0_2127e/1 -> Product_3ef8a/2
  Divide_67709/1 -> Add_f75dd/1
  Divide_0cd8d/1 -> Add_f75dd/2
  Product_eccf3/1 -> Add_fcdb9/1
  Product_30f4f/1 -> Add_fcdb9/2
  Product_3ef8a/1 -> Product_5a295/1
  Add_f75dd/1 -> Product_5a295/2
  Add_fcdb9/1 -> Subtract_4fc82/1
  Product_5a295/1 -> Subtract_4fc82/2
  Constant_2.0_47047/1 -> Product_8afa9/1
  Constant_H_bef7b/1 -> Product_8afa9/2
  Subtract_4fc82/1 -> Divide_2b866/1
  Product_8afa9/1 -> Divide_2b866/2
  Divide_2b866/1 -> Blockout_d_w_SG_D_2_78b05/1

== system IEEE14_case/SG_D_2/i_d_SG_D_2_block ==
  note: i_d_SG_D_2 in case14gfl
      | $\frac{\sin\left(\theta _{\mathrm{SG},D,2}\right)\,\left(\frac{\psi _{\mathrm{1d},\mathrm{SG},D,2}\,\left(x_{\mathrm{dd}}-x_{\mathrm{ddd}}\right)}{x_{\mathrm{dd}}-x_{l}}-\psi _{d,\mathrm{SG},D,2}+\frac{\psi _{\mathrm{fd},\mathrm{SG},D,2}\,\left(x_{\mathrm{ddd}}-x_{l}\right)}{x_{\mathrm{dd}}-x_{l}}\right)}{x_{\mathrm{ddd}}}-\frac{\cos\left(\theta _{\mathrm{SG},D,2}\right)\,\left(\psi _{q,\mathrm{SG},D,2}+\frac{\psi _{\mathrm{gq},\mathrm{SG},D,2}\,\left(x_{l}-x_{\mathrm{qdd}}\right)}{x_{l}-x_{\mathrm{qd}}}+\frac{\psi _{\mathrm{kq},\mathrm{SG},D,2}\,\left(x_{\mathrm{qd}}-x_{\mathrm{qdd}}\right)}{x_{l}-x_{\mathrm{qd}}}\right)}{x_{\mathrm{qdd}}}$
      | Automatically generated on 2025-10-09 21:31:31 .
  State_psi_gq_SG_D_2_24483 : Inport
  State_psi_kq_SG_D_2_eeb5f : Inport  Port=2
  State_psi_q_SG_D_2_b30b5 : Inport  Port=3
  State_theta_SG_D_2_acd34 : Inport  Port=4
  State_psi_1d_SG_D_2_9c394 : Inport  Port=5
  State_psi_d_SG_D_2_21b88 : Inport  Port=6
  State_psi_fd_SG_D_2_34aa6 : Inport  Port=7
  State_theta_SG_D_2_fc4e1 : Inport  Port=8
  Add_0ab75 : Sum
  Add_2ae29 : Sum
  Add_43715 : Sum
  Add_bca19 : Sum
  Add_fa741 : Sum
  Constant_-1_0644f : Constant  Value=-1
  Constant_-1_1d5d9 : Constant  Value=-1
  Constant_-1_6f1f8 : Constant  Value=-1
  Constant_-1_a0540 : Constant  Value=-1
  Constant_-1_bf8cd : Constant  Value=-1
  Constant_x_dd_072c9 : Constant  Value=x_dd
  Constant_x_dd_3f3b6 : Constant  Value=x_dd
  Constant_x_dd_61d53 : Constant  Value=x_dd
  Constant_x_ddd_62e33 : Constant  Value=x_ddd
  Constant_x_ddd_b985f : Constant  Value=x_ddd
  Constant_x_ddd_be140 : Constant  Value=x_ddd
  Constant_x_l_1a7d7 : Constant  Value=x_l
  Constant_x_l_2d345 : Constant  Value=x_l
  Constant_x_l_579e7 : Constant  Value=x_l
  Constant_x_l_a3d38 : Constant  Value=x_l
  Constant_x_l_c61e8 : Constant  Value=x_l
  Constant_x_l_c9fd7 : Constant  Value=x_l
  Constant_x_qd_571b8 : Constant  Value=x_qd
  Constant_x_qd_6bf3a : Constant  Value=x_qd
  Constant_x_qd_d9601 : Constant  Value=x_qd
  Constant_x_qdd_12781 : Constant  Value=x_qdd
  Constant_x_qdd_7e6e8 : Constant  Value=x_qdd
  Constant_x_qdd_84e98 : Constant  Value=x_qdd
  Divide_19d0e : Product  Inputs=*/
  Divide_2f6fd : Product  Inputs=*/
  Divide_4f0bb : Product  Inputs=*/
  Divide_77f71 : Product  Inputs=*/
  Divide_d7a3f : Product  Inputs=*/
  Divide_e2c18 : Product  Inputs=*/
  MathFunc_cos_4ae9d : Trigonometry  Operator=cos
  MathFunc_sin_6e229 : Trigonometry
  Product_3ef35 : Product
  Product_6c1db : Product
  Product_71349 : Product
  Product_84311 : Product
  Product_9ea1c : Product
  Product_a5169 : Product
  Product_a6c3a : Product
  Product_bea3b : Product
  Product_c9fd9 : Product
  Product_e48b7 : Product
  Product_ed9fd : Product
  Subtract_117c4 : Sum  Inputs=+-
  Subtract_4f585 : Sum  Inputs=+-
  Subtract_6445b : Sum  Inputs=+-
  Subtract_78959 : Sum  Inputs=+-
  Subtract_b6553 : Sum  Inputs=+-
  Subtract_d716a : Sum  Inputs=+-
  Subtract_e2db0 : Sum  Inputs=+-
  Subtract_f34f9 : Sum  Inputs=+-
  Blockout_i_d_SG_D_2_ab50a : Outport
  wires:
  Constant_x_ddd_be140/1 -> Subtract_f34f9/1
  Constant_x_qd_d9601/1 -> Subtract_b6553/1
  Constant_-1_a0540/1 -> Product_ed9fd/1
  Constant_-1_0644f/1 -> Product_a6c3a/1
  Subtract_117c4/1 -> Blockout_i_d_SG_D_2_ab50a/1
  Constant_x_qdd_7e6e8/1 -> Subtract_b6553/2
  Constant_x_l_1a7d7/1 -> Product_ed9fd/2
  Constant_x_l_c61e8/1 -> Product_a6c3a/2
  Product_ed9fd/1 -> Add_0ab75/1
  Product_a6c3a/1 -> Add_bca19/1
  Constant_x_l_2d345/1 -> Product_c9fd9/2
  Constant_x_qd_571b8/1 -> Add_0ab75/2
  Constant_x_qdd_84e98/1 -> Add_bca19/2
  Constant_x_qdd_12781/1 -> Divide_2f6fd/2
  MathFunc_cos_4ae9d/1 -> Product_84311/2
  Constant_-1_bf8cd/1 -> Product_c9fd9/1
  State_psi_gq_SG_D_2_24483/1 -> Product_bea3b/1
  Subtract_f34f9/1 -> Product_6c1db/2
  Product_a5169/1 -> Product_e48b7/1
  Add_0ab75/1 -> Divide_19d0e/2
  Add_bca19/1 -> Product_bea3b/2
  Product_6c1db/1 -> Divide_4f0bb/1
  Product_c9fd9/1 -> Add_fa741/1
  Constant_x_qd_6bf3a/1 -> Add_fa741/2
  State_theta_SG_D_2_fc4e1/1 -> MathFunc_sin_6e229/1
  State_psi_kq_SG_D_2_eeb5f/1 -> Product_9ea1c/1
  Add_43715/1 -> Subtract_e2db0/1
  Subtract_b6553/1 -> Product_9ea1c/2
  Product_bea3b/1 -> Divide_d7a3f/1
  Constant_-1_6f1f8/1 -> Product_a5169/1
  State_psi_1d_SG_D_2_9c394/1 -> Product_a5169/2
  State_psi_fd_SG_D_2_34aa6/1 -> Product_6c1db/1
  Constant_x_dd_61d53/1 -> Subtract_78959/1
  Product_e48b7/1 -> Divide_e2c18/1
  Constant_x_ddd_62e33/1 -> Subtract_78959/2
  Divide_4f0bb/1 -> Subtract_e2db0/2
  Add_fa741/1 -> Divide_d7a3f/2
  Product_71349/1 -> Divide_77f71/1
  Product_9ea1c/1 -> Divide_19d0e/1
  Constant_-1_1d5d9/1 -> Product_3ef35/1
  Subtract_4f585/1 -> Divide_4f0bb/2
  Subtract_78959/1 -> Product_e48b7/2
  Constant_x_dd_3f3b6/1 -> Subtract_6445b/1
  Subtract_e2db0/1 -> Product_71349/1
  Constant_x_l_a3d38/1 -> Subtract_6445b/2
  Constant_x_l_c9fd7/1 -> Subtract_f34f9/2
  Divide_d7a3f/1 -> Subtract_d716a/1
  Divide_77f71/1 -> Subtract_117c4/2
  Divide_19d0e/1 -> Subtract_d716a/2
  Subtract_6445b/1 -> Divide_e2c18/2
  Constant_x_dd_072c9/1 -> Subtract_4f585/1
  Divide_2f6fd/1 -> Subtract_117c4/1
  Constant_x_l_579e7/1 -> Subtract_4f585/2
  Subtract_d716a/1 -> Add_2ae29/1
  State_psi_q_SG_D_2_b30b5/1 -> Add_2ae29/2
  Constant_x_ddd_b985f/1 -> Divide_77f71/2
  MathFunc_sin_6e229/1 -> Product_71349/2
  Divide_e2c18/1 -> Add_43715/1
  State_psi_d_SG_D_2_21b88/1 -> Add_43715/2
  Add_2ae29/1 -> Product_3ef35/2
  State_theta_SG_D_2_acd34/1 -> MathFunc_cos_4ae9d/1
  Product_3ef35/1 -> Product_84311/1
  Product_84311/1 -> Divide_2f6fd/1
